simulink model "controller"  (R2023b)
settings: Solver=ode45  StartTime=0.0  StopTime=3  FixedStep=T  MaxStep=0.01  RelTol=1e-12  AbsTol=1e-12  EnableMultiTasking=on
values from neighbouring files (symbols this model uses):
  D = zpk(zD, pD, kD, T)    [iop_control_design_integrator.m]
  T = 0.24    [Albert.mat]    (also in D_outer_640ms.mat = 0.64; NEW_nov_11_ctrl.mat; WORKING_BACKUP.mat = 0.36; iop_control_design_integrator.m)
undefined symbols (not defined in the file or in its folder): pole, zero
libraries: cstblocks x2
settings Model: Creator=cnielsen  LastModifiedBy=lucs1
settings SolverCC: AutoScaleAbsTol=off  AlgebraicLoopSolver=TrustRegion
settings DataIOCC: SaveFormat=Array  SignalLoggingSaveFormat=ModelDataLogs  SaveOutput=off  SaveTime=off  ReturnWorkspaceOutputs=off  Refine=5
settings OptimizationCC: ExpressionDepthLimit=2147483647  LifeSpan=inf
settings DebuggingCC: UnderspecifiedInitializationDetection=Classic  MergeDetectMultiDrivingBlocksExec=none  SolverPrmCheckMsg=warning  FcnCallInpInsideContextMsg=warning  UnconnectedInputMsg=warning  UnconnectedOutputMsg=warning  UnconnectedLineMsg=warning  StateNameClashWarn=warning  SFUnexpectedBacktrackingDiag=warning  SFNoUnconditionalDefaultTransitionDiag=warning  SFExecutionAtInitializationDiag=none  ArithmeticOperatorsInVariantConditions=warning
settings HardwareCC: ProdBitPerPointer=32  ProdBitPerSizeT=32  ProdBitPerPtrDiffT=32  ProdLargestAtomicFloat=None  ProdIntDivRoundTo=Undefined  ProdEndianess=Unspecified  ProdWordSize=32  ProdHWDeviceType=32-bit Generic
settings ModelReferenceCC: PropagateSignalLabelsOutOfModel=off
settings SFSimCC: SimUseLocalCustomCode=off  CustomCodeUndefinedFunction=UseInterfaceOnly
settings RTWCC: RTWUseLocalCustomCode=off
settings CodeAppCC: StateflowObjectComments=on
settings GRTTargetCC: TargetLangStandard=C89/C90 (ANSI)  CombineOutputUpdateFcns=off  GRTInterface=on
settings ConfigComp: CovMetricSettings=dw  CovSaveCumulativeToWorkspaceVar=on  CovSaveSingleToWorkspaceVar=on  CovExternalEMLEnable=off

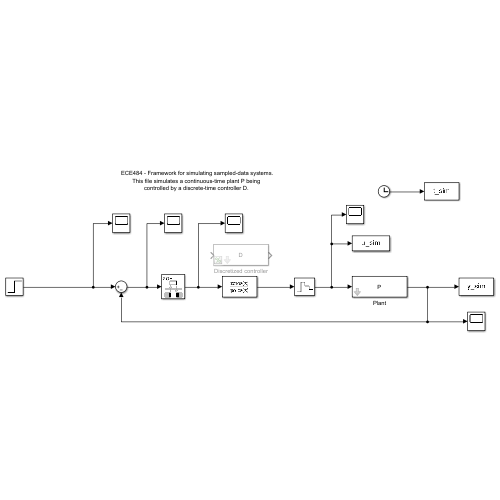
[thumbnail: Simulink's stored preview of the top-level diagram]
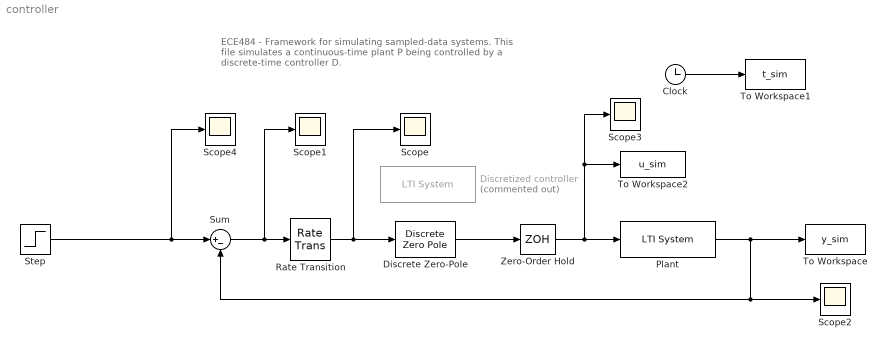
== system controller ==
  note: ECE484 - Framework for simulating sampled-data systems.
      | This file simulates a continuous-time plant P being
      | controlled by a discrete-time controller D.
  Clock : Clock
  Discrete Zero-Pole : DiscreteZeroPole  Zeros=zero(D)  Poles=pole(D)  Gain=D.K  SampleTime=D.Ts
  Discretized controller : cstblocks/LTI System  Commented=on  sys=D  IC=[]  PadeOrder=0
  Plant : cstblocks/LTI System  sys=P  IC=[]  PadeOrder=0
  Rate Transition : RateTransition  OutPortSampleTime=T
  Scope{,1..4} (5 alike) : Scope
  Step : Step  Time=0  After=1.4  SampleTime=T
  Sum : Sum  Inputs=|+-
  To Workspace : ToWorkspace  VariableName=y_sim  SampleTime=-1
  To Workspace1 : ToWorkspace  VariableName=t_sim  SampleTime=-1
  To Workspace2 : ToWorkspace  VariableName=u_sim
  Zero-Order Hold : ZeroOrderHold  SampleTime=D.Ts
  wires:
  Clock/1 -> To Workspace1/1
  Step/1 -> Scope4/1, Sum/1
  Plant/1 -> To Workspace/1, Sum/2, Scope2/1
  Sum/1 -> Rate Transition/1, Scope1/1
  Discrete Zero-Pole/1 -> Zero-Order Hold/1
  Rate Transition/1 -> Discrete Zero-Pole/1, Scope/1
  Zero-Order Hold/1 -> Plant/1, Scope3/1, To Workspace2/1
